simulink model "robot_and_motors"  (R2018a)
settings: Solver=ode45  StartTime=0.0  StopTime=4  FixedStep=0.005  RelTol=1e-3  EnableMultiTasking=on
values from neighbouring files (symbols this model uses):
  robot = load_robot('example', '2dofplanar')    [motor_selection_2dofplanar.m]
undefined symbols (not defined in the file or in its folder): call_direct_dynamics_2dofplanar_s3b
settings Model: Creator=arturo  LastModifiedBy=arturogilaparicio
settings DataIOCC: SaveFormat=Array  SignalLoggingSaveFormat=ModelDataLogs
settings OptimizationCC: ExpressionDepthLimit=2147483647  LifeSpan=inf
settings DebuggingCC: UnderspecifiedInitializationDetection=Classic  MergeDetectMultiDrivingBlocksExec=none  SolverPrmCheckMsg=warning  FcnCallInpInsideContextMsg=warning  StateNameClashWarn=warning  SFUnexpectedBacktrackingDiag=warning  SFNoUnconditionalDefaultTransitionDiag=warning  SFExecutionAtInitializationDiag=none
settings HardwareCC: ProdBitPerPointer=32  ProdBitPerSizeT=32  ProdBitPerPtrDiffT=32  ProdLargestAtomicFloat=None  ProdIntDivRoundTo=Undefined  ProdEndianess=Unspecified  ProdWordSize=32  ProdHWDeviceType=32-bit Generic
settings ModelReferenceCC: PropagateSignalLabelsOutOfModel=off
settings SFSimCC: SimParseCustomCode=off
settings CodeAppCC: StateflowObjectComments=on
settings GRTTargetCC: TargetLangStandard=C89/C90 (ANSI)  GeneratePreprocessorConditionals=Disable all  CombineOutputUpdateFcns=off  GRTInterface=on
settings ConfigComp: CovMetricSettings=dw  CovHtmlReporting=on  CovSaveCumulativeToWorkspaceVar=on  CovSaveSingleToWorkspaceVar=on  CovExternalEMLEnable=off

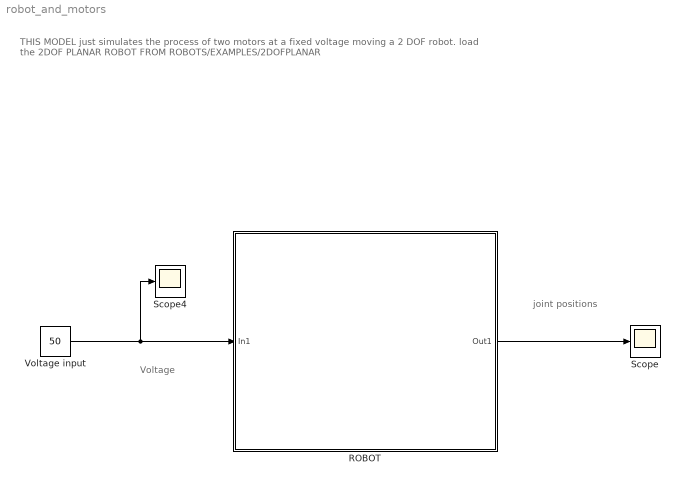
== system robot_and_motors ==
  note: THIS MODEL just simulates the process of two motors at a fixed voltage moving a 2 DOF robot.
      |
      | load the 	2DOF PLANAR ROBOT FROM ROBOTS/EXAMPLES/2DOFPLANAR
  note: Voltage
  note: joint positions
  ROBOT : Subsystem
      mask Display: image(imread('images/robot2dof.png'))
  Scope : Scope
  Scope4 : Scope
  "Voltage input " : Constant  Value=50
  wires:
  "Voltage input "/1 -> ROBOT/1(In1), Scope4/1
  ROBOT/1(Out1) -> Scope/1

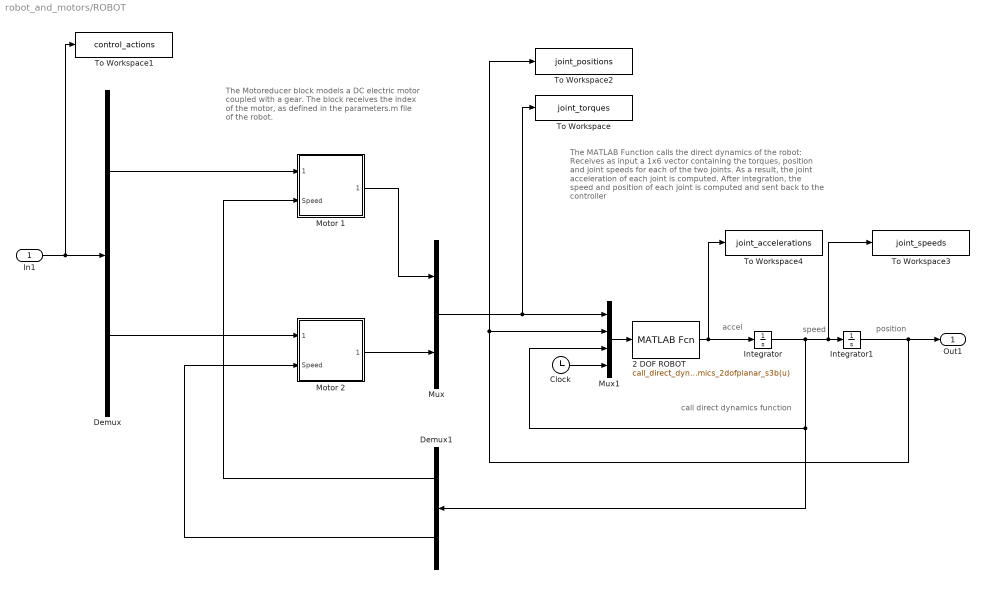
== system robot_and_motors/ROBOT ==
  note: accel
  note: speed
  note: position
  note: The MATLAB Function calls the direct dynamics of the robot:
      | Receives as input a 1x6 vector containing the
      | torques, position and joint
      | speeds for each of the two joints. As a result, the joint
      | acceleration of each joint is computed.
      | After integration, the speed and position of each joint
      | is computed and sent back to the controller
  note: call direct dynamics
      |  function
  note: The Motoreducer block models a DC
      | electric motor coupled with a gear.
      | The block receives the index of the motor,
      | as defined in the parameters.m file of the robot.
  In1 : Inport
  2 DOF ROBOT : MATLABFcn  MATLABFcn=call_direct_dynamics_2dofplanar_s3b(u)  OutputDimensions=2
  Clock : Clock
  Demux : Demux  Outputs=2
  Demux1 : Demux  Outputs=2
  Integrator : Integrator  InitialCondition=[0 0 ]
  Integrator1 : Integrator  InitialCondition=[0 0]
  Motor 1 : Subsystem
  Motor 2 : Subsystem
  Mux : Mux  Inputs=2
  Mux1 : Mux
  To Workspace : ToWorkspace  VariableName=joint_torques  SampleTime=-1
  To Workspace1 : ToWorkspace  VariableName=control_actions  SampleTime=-1
  To Workspace2 : ToWorkspace  VariableName=joint_positions  SampleTime=-1
  To Workspace3 : ToWorkspace  VariableName=joint_speeds  SampleTime=-1
  To Workspace4 : ToWorkspace  VariableName=joint_accelerations  SampleTime=-1
  Out1 : Outport
  wires:
  Demux/1 -> Motor 1/1(Input (Volts))
  Demux/2 -> Motor 2/1(Input (Volts))
  Mux1/1 -> 2 DOF ROBOT/1
  2 DOF ROBOT/1 -> To Workspace4/1, Integrator/1
  Integrator/1 -> To Workspace3/1, Integrator1/1, Demux1/1, Mux1/3
  Motor 1/1(Output Torque) -> Mux/1
  Demux1/1 -> Motor 1/2(Speed)
  Motor 2/1(Output Torque) -> Mux/2
  Demux1/2 -> Motor 2/2(Speed)
  In1/1 -> To Workspace1/1, Demux/1
  Integrator1/1 -> Out1/1, Mux1/2, To Workspace2/1
  Mux/1 -> Mux1/1, To Workspace/1
  Clock/1 -> Mux1/4

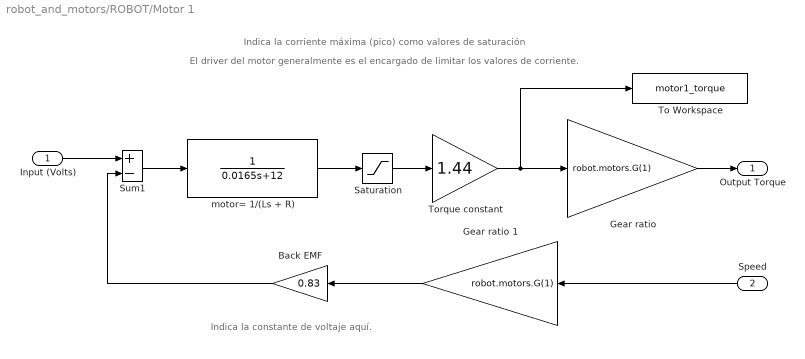
== system robot_and_motors/ROBOT/Motor 1 ==
  note: Indica la constante de voltaje aquí.
  note: El driver del motor generalmente es el encargado de limitar los valores de corriente.
  note: Indica la corriente máxima (pico) como valores de saturación
  Input (Volts) : Inport
  Speed : Inport  Port=2
  Back EMF : Gain  Gain=0.83  SaturateOnIntegerOverflow=on  OutDataTypeStr=Inherit: Same as input  ParamDataTypeStr=Inherit: Same as input
  Gear ratio : Gain  Gain=robot.motors.G(1)  SaturateOnIntegerOverflow=on  OutDataTypeStr=Inherit: Same as input  ParamDataTypeStr=Inherit: Same as input
  Gear ratio 1 : Gain  Gain=robot.motors.G(1)  SaturateOnIntegerOverflow=on  OutDataTypeStr=Inherit: Same as input  ParamDataTypeStr=Inherit: Same as input
  Saturation : Saturate  UpperLimit=11  LowerLimit=-11  ZeroCross=off
  Sum1 : Sum  Inputs=+-  SaturateOnIntegerOverflow=on  InputSameDT=on  OutDataTypeStr=Inherit: Same as first input
  To Workspace : ToWorkspace  VariableName=motor1_torque  SampleTime=-1
  Torque constant : Gain  Gain=1.44  SaturateOnIntegerOverflow=on  OutDataTypeStr=Inherit: Same as input  ParamDataTypeStr=Inherit: Same as input
  motor= 1/(Ls + R) : TransferFcn  Denominator=[0.0165 12]
  Output Torque : Outport  InitialOutput=0
  wires:
  Gear ratio 1/1 -> Back EMF/1
  Speed/1 -> Gear ratio 1/1
  Input (Volts)/1 -> Sum1/1
  Back EMF/1 -> Sum1/2
  Sum1/1 -> motor= 1/(Ls + R)/1
  Gear ratio/1 -> Output Torque/1
  Torque constant/1 -> To Workspace/1, Gear ratio/1
  motor= 1/(Ls + R)/1 -> Saturation/1
  Saturation/1 -> Torque constant/1

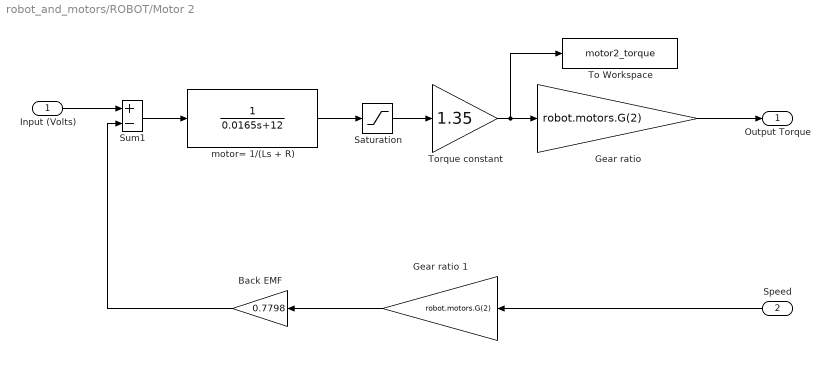
== system robot_and_motors/ROBOT/Motor 2 ==
  Input (Volts) : Inport
  Speed : Inport  Port=2
  Back EMF : Gain  Gain=0.7798  SaturateOnIntegerOverflow=on  OutDataTypeStr=Inherit: Same as input  ParamDataTypeStr=Inherit: Same as input
  Gear ratio : Gain  Gain=robot.motors.G(2)  SaturateOnIntegerOverflow=on  OutDataTypeStr=Inherit: Same as input  ParamDataTypeStr=Inherit: Same as input
  Gear ratio 1 : Gain  Gain=robot.motors.G(2)  SaturateOnIntegerOverflow=on  OutDataTypeStr=Inherit: Same as input  ParamDataTypeStr=Inherit: Same as input
  Saturation : Saturate  UpperLimit=9  LowerLimit=-9  ZeroCross=off
  Sum1 : Sum  Inputs=+-  SaturateOnIntegerOverflow=on  InputSameDT=on  OutDataTypeStr=Inherit: Same as first input
  To Workspace : ToWorkspace  VariableName=motor2_torque  SampleTime=-1
  Torque constant : Gain  Gain=1.35  SaturateOnIntegerOverflow=on  OutDataTypeStr=Inherit: Same as input  ParamDataTypeStr=Inherit: Same as input
  motor= 1/(Ls + R) : TransferFcn  Denominator=[0.0165 12]
  Output Torque : Outport  InitialOutput=0
  wires:
  Saturation/1 -> Torque constant/1
  motor= 1/(Ls + R)/1 -> Saturation/1
  Torque constant/1 -> To Workspace/1, Gear ratio/1
  Gear ratio/1 -> Output Torque/1
  Sum1/1 -> motor= 1/(Ls + R)/1
  Back EMF/1 -> Sum1/2
  Input (Volts)/1 -> Sum1/1
  Speed/1 -> Gear ratio 1/1
  Gear ratio 1/1 -> Back EMF/1
